simulink model "EarlyReturn15"  (R2020a)
settings: Solver=VariableStepAuto  StartTime=0.0  StopTime=0.1  RelTol=1e-3
settings Model: Creator=BEAR  LastModifiedBy=bzhan
settings DataIOCC: ReturnWorkspaceOutputs=off
settings DebuggingCC: ArithmeticOperatorsInVariantConditions=warning
settings SFSimCC: SimUseLocalCustomCode=off  CustomCodeUndefinedFunction=UseInterfaceOnly
settings RTWCC: RTWUseLocalCustomCode=off

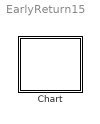
== system EarlyReturn15 ==
  Chart : Stateflow chart  TreatAsAtomicUnit=on

== stateflow chart EarlyReturn15/Chart ==
  state S
    en: f("enS")
    state A1 [parallel]
      en: f("enA1_start");
      E;f("enA1_done")
      settings: executionOrder=1
    state A2 [parallel]
      en: f("enA2")
      settings: executionOrder=2
  state B
    en: f("enB")
  state C
    en: f("enC")
  (default) -> S
  S -> B : E
  B -> C
  data: s function_input
  events: E local FUNCTION_CALL_EVENT
  function f(s):
    | function f(s)
    |   fprintf(s+"\n");
